simulink library "bat_lib"  (R2026a)
settings: Solver=VariableStepAuto
libraries: fl_lib x11, nesl_utility x5

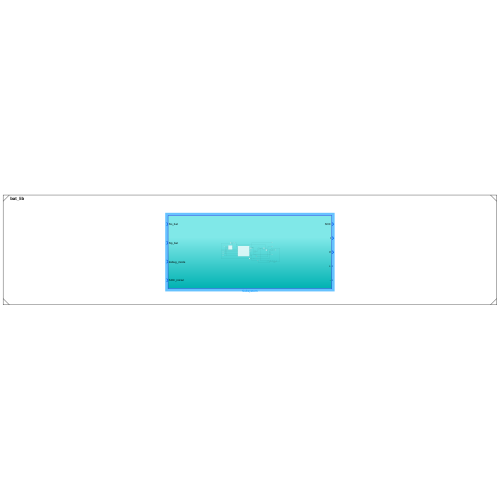
[thumbnail: Simulink's stored preview of the top-level diagram]
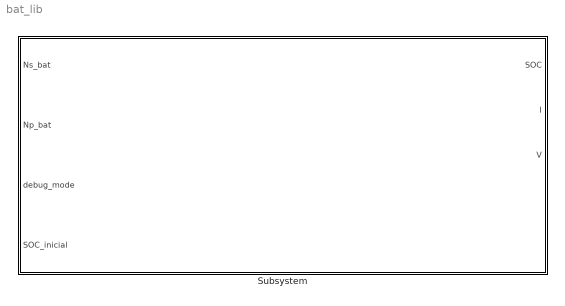
== system bat_lib ==
  Subsystem : Subsystem

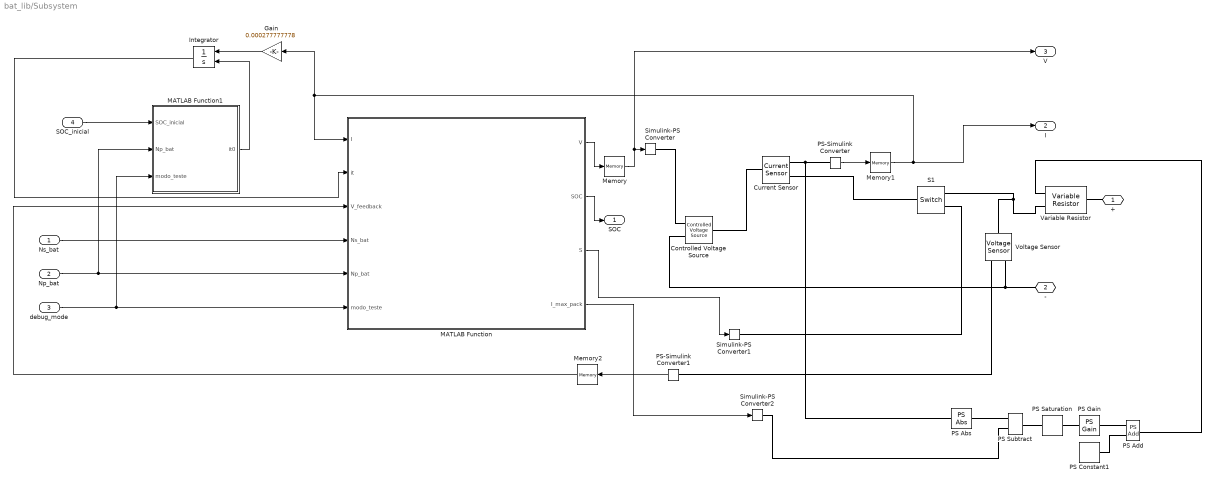
== system bat_lib/Subsystem ==
  Ns_bat : Inport
  Np_bat : Inport  Port=2
  debug_mode : Inport  Port=3
  SOC_inicial : Inport  Port=4
  Controlled Voltage Source : fl_lib/Electrical/Electrical Sources/Controlled Voltage Source
  Current Sensor : fl_lib/Electrical/Electrical Sensors/Current Sensor
  Gain : Gain  Gain=0.000277777778
  Integrator : Integrator  InitialConditionSource=external
  MATLAB Function : MATLAB Function  TreatAsAtomicUnit=on
  MATLAB Function1 : MATLAB Function  TreatAsAtomicUnit=on
  Memory : Memory
  Memory1 : Memory
  Memory2 : Memory
  PS Abs : fl_lib/Physical Signals/Nonlinear Operators/PS Abs  ZeroCross=true
  PS Add : fl_lib/Physical Signals/Functions/PS Add
  PS Constant1 : fl_lib/Physical Signals/Sources/PS Constant  constant=0.001 Ohm
  PS Gain : fl_lib/Physical Signals/Functions/PS Gain  gain=50 Ohm/A
  PS Saturation : fl_lib/Physical Signals/Nonlinear Operators/PS Saturation  upper_limit=100000 A  lower_limit=0 A  ZeroCross=true
  PS Subtract : fl_lib/Physical Signals/Functions/PS Subtract
  PS-Simulink Converter : nesl_utility/PS-Simulink Converter  PhysicalDomain=network_engine_domain  SubClassName=ps_output  LeftPortType=input  RightPortType=output  PseudoPeriodic=off  Frequencies=[]  VectorFormat=inherit  Unit=inherit  AffineConversion=off
  PS-Simulink Converter1 : nesl_utility/PS-Simulink Converter  PhysicalDomain=network_engine_domain  SubClassName=ps_output  LeftPortType=input  RightPortType=output  PseudoPeriodic=off  Frequencies=[]  VectorFormat=inherit  Unit=inherit  AffineConversion=off
  S1 : fl_lib/Electrical/Electrical Elements/Switch  R_closed=.001 Ohm  G_open=1e-6 1/Ohm  Threshold=0.5  i_specify=off  i_priority=None  i=0 A  i_nominal_specify=off  i_nominal_value=1  i_nominal_unit=A  v_specify=off  v_priority=None  v=0 V  v_nominal_specify=off  v_nominal_value=1  v_nominal_unit=V
  Simulink-PS Converter : nesl_utility/Simulink-PS Converter  PhysicalDomain=network_engine_domain  SubClassName=ps_input  LeftPortType=input  RightPortType=output  PseudoPeriodic=off  Frequencies=[]  NoiseDistribution=none  NoiseParameters=[]  Unit=1  AffineConversion=off  FilteringAndDerivatives=provide  SimscapeFilterOrder=1  InputFilterTimeConstant=0.001  UdotUserProvided=0
  Simulink-PS Converter1 : nesl_utility/Simulink-PS Converter  PhysicalDomain=network_engine_domain  SubClassName=ps_input  LeftPortType=input  RightPortType=output  PseudoPeriodic=off  Frequencies=[]  NoiseDistribution=none  NoiseParameters=[]  Unit=1  AffineConversion=off  FilteringAndDerivatives=provide  SimscapeFilterOrder=1  InputFilterTimeConstant=0.001  UdotUserProvided=0
  Simulink-PS Converter2 : nesl_utility/Simulink-PS Converter  PhysicalDomain=network_engine_domain  SubClassName=ps_input  LeftPortType=input  RightPortType=output  PseudoPeriodic=off  Frequencies=[]  NoiseDistribution=none  NoiseParameters=[]  Unit=A  AffineConversion=off  FilteringAndDerivatives=provide  SimscapeFilterOrder=1  InputFilterTimeConstant=0.001  UdotUserProvided=0
  Variable Resistor : fl_lib/Electrical/Electrical Elements/Variable Resistor  Rmin=0 Ohm  thermalEnable=false  thermal_mass=1 J/K  i_specify=off  i_priority=None  i=0 A  i_nominal_specify=off  i_nominal_value=1  i_nominal_unit=A  v_specify=off  v_priority=None  v=0 V  v_nominal_specify=off  v_nominal_value=1  v_nominal_unit=V  T_specify=off  T_priority=None  T=300 K  T_nominal_specify=off  T_nominal_value=1  T_nominal_unit=K
  Voltage Sensor : fl_lib/Electrical/Electrical Sensors/Voltage Sensor
  + : PMIOPort  Side=Right
  - : PMIOPort  Port=2  Side=Right
  SOC : Outport
  I : Outport  Port=2
  V : Outport  Port=3
  wires:
  Gain/1 -> Integrator/1
  MATLAB Function/2(SOC) -> SOC/1
  Integrator/1 -> MATLAB Function/2(it)
  MATLAB Function/1(V) -> Memory/1
  Memory/1 -> V/1, Simulink-PS Converter/1
  PS-Simulink Converter/1 -> Memory1/1
  Memory1/1 -> MATLAB Function/1(I), Gain/1, I/1
  MATLAB Function/3(S) -> Simulink-PS Converter1/1
  PS-Simulink Converter1/1 -> Memory2/1
  Memory2/1 -> MATLAB Function/3(V_feedback)
  MATLAB Function/4(I_max_pack) -> Simulink-PS Converter2/1
  debug_mode/1 -> MATLAB Function1/3(modo_teste), MATLAB Function/6(modo_teste)
  Np_bat/1 -> MATLAB Function1/2(Np_bat), MATLAB Function/5(Np_bat)
  Ns_bat/1 -> MATLAB Function/4(Ns_bat)
  MATLAB Function1/1(it0) -> Integrator/2
  SOC_inicial/1 -> MATLAB Function1/1(SOC_inicial)
  connections:
  Controlled Voltage Source/RConn2 -- Voltage Sensor/RConn2 -- -/RConn1
  PS-Simulink Converter/LConn1 -- PS Abs/LConn1 -- Current Sensor/RConn1
  Simulink-PS Converter/RConn1 -- Controlled Voltage Source/RConn1
  Controlled Voltage Source/LConn1 -- Current Sensor/LConn1
  S1/LConn1 -- Current Sensor/RConn2
  S1/RConn2 -- Voltage Sensor/LConn1 -- Variable Resistor/LConn2
  Simulink-PS Converter1/RConn1 -- S1/RConn1
  Voltage Sensor/RConn1 -- PS-Simulink Converter1/LConn1
  Variable Resistor/RConn1 -- +/RConn1
  Simulink-PS Converter2/RConn1 -- PS Subtract/LConn2
  PS Abs/RConn1 -- PS Subtract/LConn1
  PS Saturation/LConn1 -- PS Subtract/RConn1
  PS Saturation/RConn1 -- PS Gain/LConn1
  PS Gain/RConn1 -- PS Add/LConn1
  PS Constant1/RConn1 -- PS Add/LConn2
  PS Add/RConn1 -- Variable Resistor/LConn1

== matlab function bat_lib/Subsystem/MATLAB Function1 ==
  data: SOC_inicial input; it0 output; Np_bat input; modo_teste input
function it0 = calc_it0(SOC_inicial, Np_bat, modo_teste)
    % Replica a mesma lógica de Q usada no modelo_bateria,
    % pra it0 ficar consistente com o Q efetivo da simulação.
    Q_1_real = 2.3;
    Q_1_teste = 0.00055;

    if modo_teste == 1
        Q_1 = Q_1_teste;
    else
        Q_1 = Q_1_real;
    end

    Q = Q_1 * Np_bat;
    it0 = Q * (1 - SOC_inicial/100);
end

== matlab function bat_lib/Subsystem/MATLAB Function ==
  data: I input; V output; it input; SOC output; S output; V_feedback input; Ns_bat input; Np_bat input; modo_teste input; I_max_pack output
function [V, SOC, S,I_max_pack] = modelo_bateria(I, it, V_feedback, Ns_bat, Np_bat, modo_teste)
    % ---- Parâmetros de UM pack (4S Li-ion genérico, valores REAIS) ----
    E0_1 = 16.8;
    Q_1_real  = 2.3;
    R_1  = 0.01;
    K_1_real  = 0.0076;
    A_1  = 0.26422;
    B_1_real  = 26.5487;
    V_max_1 = 19.0;
    V_min_1 = 13.5;
    margem_religa_1 = 0.3
    C = 2.3; % Taxa de descarga de 2.3A
    I_max_desc = C * 2;
    I_max_carga = C *  0.5;
    % ---- Modo teste: encolhe Q (e escala K, B pelo mesmo fator) ----
    % para ver a curva de carga/descarga em segundos em vez de horas.
    % A NÃO escala. NUNCA usar modo_teste=1 para resultado final.
    if modo_teste == 1
        Q_1 = 0.00055;
        f = Q_1_real / Q_1;
        K_1 = K_1_real * f;
        B_1 = B_1_real * f;
    else
        Q_1 = Q_1_real;
        K_1 = K_1_real;
        B_1 = B_1_real;
    end

    % ---- Escala pro banco (Ns_bat em série, Np_bat em paralelo) ----
    E0 = E0_1 * Ns_bat;
    Q  = Q_1  * Np_bat;
    R  = R_1  * Ns_bat / Np_bat;
    K  = K_1  * Ns_bat;
    A  = A_1  * Ns_bat;
    B  = B_1  / Np_bat;
    V_max = V_max_1 * Ns_bat;
    V_min = V_min_1 * Ns_bat;
    margem_religa = margem_religa_1 * Ns_bat;

    if I < 0
        I_max_pack = I_max_carga * Np_bat;
    else
        I_max_pack = I_max_desc * Np_bat;
    end

    it_c = min(max(it, 0), 0.99*Q);
    E = E0 - K*(Q/(Q - it_c))*it_c + A*exp(-B*it_c);
    V = E - I*R;
    SOC = 100*(1 - it/Q);
    if SOC < 0
        SOC = 0;
    elseif SOC > 100
        SOC = 100;
    end
    % --- Lógica de proteção/religamento ---
    if V < V_min || SOC <= 0
        if V_feedback > (E + margem_religa)
            S = 1;
        else
            S = 0;
        end
    elseif V > V_max
        S = 0;
    elseif SOC >= 100 && I < 0
        S = 0;   % bloqueia carga quando já está cheia
    else
        S = 1;
    end
    if V < V_min
        V = V_min;
    elseif V > V_max
        V = V_max;
    end
end
